simulink model "receiver"  (R2021b)
settings: Solver=VariableStepAuto  StartTime=0.0  StopTime=10000/3.2e6  RelTol=1e-3
PreLoadFcn:
  | setup_receiver
InitFcn:
  | setup_receiver
values from neighbouring files (symbols this model uses):
  fir_bbuf = reshape([fir_barker_13; fir_barker_13; fir_barker_13], [1, length(fir_barker_13)*3])    [setup_receiver.m]
  tx_data = [tx_data mbuf]    [setup_receiver.m]
undefined symbols (not defined in the file or in its folder): AXI4, designMultirateFIR, Lite, xlfda_numerator
libraries: hdlBasic x467, hdlsllib x15, dspmlti4 x8, hdlDSPIP x6, hdlSSR x6, dspswit3 x4, hdlUtilities x3, commrandsrc3 x2, dspsigops x2, simulink x1, vmcUtilities x1
(part 4 of 6)

== system receiver/QPSK System/RF-DAC ==
  note: Not Ready
  Data In : Inport
  Coarse Delay : Subsystem
  Interpolation Filter : Subsystem  mask{interp=8x}
      mask prompts: interp "Interpolation Factor:"
      mask init:
      | fir0 = dsp.FIRInterpolator('InterpolationFactor', 2,...
      |                            'CoefficientsDataType', 'Custom',...
      |                            'CustomCoefficientsDataType', numerictype([], 16, 14),...
      |                            'FullPrecisionOverride', false,...
      |                            'OutputDataType', 'Custom',...
      |                            'CustomOutputDataType', numerictype([], 16, 14),...
      |                            'Numerator', [-6, 0 54, 0, -254, 0, 1230, 2048, 1230, 0, -254, 0, 54, 0, -6]/(2048));
      | fir1 = dsp.FIRInterpolator('InterpolationFactor', 2,...
      |                            'CoefficientsDataType', 'Custom',...
      |                            'CustomCoefficientsDataType', numerictype([], 16, 14),...
      |                            'FullPrecisionOverride', false,...
      |                            'OutputDataType', 'Custom',...
      |                            'CustomOutputDataType', numerictype([], 16, 14),...
      |                            'Numerator', [-12, 0, 84, 0, -337, 0, 1008, 0, -2693, 0, 10142, 16384, 10142, 0, -2693, 0, 1008, 0, -337, 0, 84, 0 ,-12]/(16384));
      | fir2 = dsp.FIRInterpolator('InterpolationFactor', 2,...
      |                            'CoefficientsDataType', 'Custom',...
      |                            'CustomCoefficientsDataType', numerictype([], 16, 14),...
      |                            'FullPrecisionOverride', false,...
      |                            'OutputDataType', 'Custom',...
      |                            'CustomOutputDataType', numerictype([], 16, 14),...
      |                            'Numerator', [5, 0, -17, 0, 44, 0, -96, 0, 187, 0, -335, 0, 565, 0, -906, 0, 1401, 0, -2112, 0, 3145, 0, -4723, 0, 7415, 0, -13331, 0, 41526, 65536, 41526, 0, -13331, 0, 7415, 0, -4723, 0, 3145, 0, -2112, 0, 1401, 0, -906, 0, 565, 0, -335, 0, 187, 0, -96, 0, 44, 0, -17, 0, 5]/(65536));
      | switch get_param(gcb, 'interp')
      |     case '1x'
      |         if ~strcmp(get_param([gcb, '/FIR 0'], 'Commented'), 'through')
      |             set_param([gcb, '/FIR 0'],'Commented','through');
      |         end
      |         
      |         if ~strcmp(get_param([gcb, '/FIR 1'], 'Commented'), 'through')
      |             set_param([gcb, '/FIR 1'],'Commented','through');
      |         end
      |         
      |         if ~strcmp(get_param([gcb, '/FIR 2'], 'Commented'), 'through')
      |             set_param([gcb, '/FIR 2'],'Commented','through');
      |         end
      |             
      |     case '2x'
      |         if ~strcmp(get_param([gcb, '/FIR 0'], 'Commented'), 'through')
      |             set_param([gcb, '/FIR 0'],'Commented','through');
      |         end
      |         
      |         if ~strcmp(get_param([gcb, '/FIR 1'], 'Commented'), 'through')
      |             set_param([gcb, '/FIR 1'],'Commented','through');
      |         end
      |         
      |         if ~strcmp(get_param([gcb, '/FIR 2'], 'Commented'), 'off')
      |             set_param([gcb, '/FIR 2'],'Commented','off');
      |         end
      | 
      |     case '4x'
      |         if ~strcmp(get_param([gcb, '/FIR 0'], 'Commented'), 'through')
      |             set_param([gcb, '/FIR 0'],'Commented','through');
      |         end
      |         
      |         if ~strcmp(get_param([gcb, '/FIR 1'], 'Commented'), 'off')
      |             set_param([gcb, '/FIR 1'],'Commented','off');
      |         end
      |         
      |         if ~strcmp(get_param([gcb, '/FIR 2'], 'Commented'), 'off')
      |             set_param([gcb, '/FIR 2'],'Commented','off');
      |         end
      |         
      |     case '8x'
      |         if ~strcmp(get_param([gcb, '/FIR 0'], 'Commented'), 'off')
      |             set_param([gcb, '/FIR 0'],'Commented','off');
      |         end
      |         
      |         if ~strcmp(get_param([gcb, '/FIR 1'], 'Commented'), 'off')
      |             set_param([gcb, '/FIR 1'],'Commented','off');
      |         end
      |         
      |         if ~strcmp(get_param([gcb, '/FIR 2'], 'Commented'), 'off')
      |             set_param([gcb, '/FIR 2'],'Commented','off');
      |         end
      | 
      | end
      mask TypeOptions interp: 1x | 2x | 4x | 8x
      mask DialogControl DescGroupVar Prompt: RF-DAC Interpolation Filter
      mask DialogControl DescTextVar Prompt: This block simulates the RF-DAC interpolation stage using the same coefficients stored in the interpolation filters.
      mask DialogControl ParameterGroupVar Prompt: Main
  NCO and Mixer : Subsystem
  Output Filter : Subsystem
  QMC Gain & Phase : Subsystem
  QMC Threshold : Subsystem
  RF-DAC : Subsystem
  Data Out : Outport  VectorParamsAs1DForOutWhenUnconnected=off
  wires:
  RF-DAC/1(Data Out) -> Data Out/1
  QMC Threshold/1(Data Out) -> RF-DAC/1(Data In)
  Output Filter/1(Data Out) -> QMC Threshold/1(Data In)
  Coarse Delay/1(Data Out) -> Output Filter/1(Data In)
  QMC Gain & Phase/1(Data Out) -> Coarse Delay/1(Data In)
  Data In/1 -> Interpolation Filter/1(Data In)
  NCO and Mixer/1(Data Out) -> QMC Gain & Phase/1(Data In)
  Interpolation Filter/1(Data Out) -> NCO and Mixer/1(Data In)

== system receiver/Time Synchronisation/Loop Filter ==
  note: Get centre of symbol
  note: The input to the loop filter should only be changed once per symbol.
      |
      | Use an enable register with the strobe from the NCC to hold the data in place.
  note: Get centre of symbol
  Real In : Inport
  Imag In : Inport  Port=2
  Signal In : Inport  Port=3
  Valid In : Inport  Port=4
  Reset : Inport  Port=5
  AddSub : hdlBasic/AddSub  mode=Addition  use_carryin=off  use_carryout=off  en=off  latency=0  precision=User Defined  arith_type="Signed  (2's comp)"  n_bits=64  bin_pt=60  quantization=Truncate  overflow=Saturate  use_behavioral_HDL=off  hw_selection=Fabric  pipelined=off  XmcBlockStatus=1  maskContainerNames=tabcontainer1  block_type=addsub  block_config=sysgen:Addsub_config
  AddSub1 : hdlBasic/AddSub  mode=Addition  use_carryin=off  use_carryout=off  en=off  latency=0  precision=User Defined  arith_type="Signed  (2's comp)"  n_bits=64  bin_pt=60  quantization=Truncate  overflow=Saturate  use_behavioral_HDL=off  hw_selection=Fabric  pipelined=off  XmcBlockStatus=1  maskContainerNames=tabcontainer1  block_type=addsub  block_config=sysgen:Addsub_config
  Delay1 : hdlBasic/Delay  rst=off  en=off  latency=32/2  reg_retiming=off  XmcBlockStatus=1  maskContainerNames=group1  block_type=delay  block_config=sysgen:Delay_config
  Delay2 : hdlBasic/Delay  rst=off  en=off  latency=32/2  reg_retiming=off  XmcBlockStatus=1  maskContainerNames=group1  block_type=delay  block_config=sysgen:Delay_config
  Delay3 : hdlBasic/Delay  rst=off  en=off  latency=32/2  reg_retiming=off  XmcBlockStatus=1  maskContainerNames=group1  block_type=delay  block_config=sysgen:Delay_config
  K1_Gain : hdlBasic/CMult  const=K1  gui_display_data_type=Fixed-point  const_n_bits=32  const_bin_pt=30  float_type=Single  exp_bits=8  fraction_bits=24  en=off  latency=0  precision=Full  arith_type="Signed  (2's comp)"  n_bits=3+28+16  bin_pt=28+16  quantization=Truncate  overflow=Wrap  use_behavioral_HDL=off  mem_type=Distributed RAM  pipeline=off  XmcBlockStatus=1  maskContainerNames=tabcontainer1  block_type=cmult  block_config=sysgen:CMult_config
      settings: infoedit=[]
  K2_Gain : hdlBasic/CMult  const=K2  gui_display_data_type=Fixed-point  const_n_bits=32  const_bin_pt=30  float_type=Single  exp_bits=8  fraction_bits=24  en=off  latency=0  precision=Full  arith_type="Signed  (2's comp)"  n_bits=3+28+16  bin_pt=28+16  quantization=Truncate  overflow=Wrap  use_behavioral_HDL=off  mem_type=Distributed RAM  pipeline=off  XmcBlockStatus=1  maskContainerNames=tabcontainer1  block_type=cmult  block_config=sysgen:CMult_config
      settings: infoedit=[]
  Register : hdlBasic/Register  init=0  rst=on  en=on  XmcBlockStatus=1  maskContainerNames=tabcontainer1  block_type=register  block_config=sysgen:Register_config
  Register1 : hdlBasic/Register  init=0  rst=on  en=on  XmcBlockStatus=1  maskContainerNames=tabcontainer1  block_type=register  block_config=sysgen:Register_config
  Real Out : Outport  VectorParamsAs1DForOutWhenUnconnected=off
  Imag Out : Outport  Port=2  VectorParamsAs1DForOutWhenUnconnected=off
  Valid Out : Outport  Port=3  VectorParamsAs1DForOutWhenUnconnected=off
  Error Out : Outport  Port=4  VectorParamsAs1DForOutWhenUnconnected=off
  wires:
  Valid In/1 -> Register1/3, Delay3/1, Register/3
  AddSub1/1 -> Error Out/1
  Delay1/1 -> Real Out/1
  Delay2/1 -> Imag Out/1
  Register1/1 -> K2_Gain/1, K1_Gain/1
  Signal In/1 -> Register1/1
  Register/1 -> AddSub/2
  K1_Gain/1 -> AddSub1/1
  AddSub/1 -> AddSub1/2, Register/1
  Imag In/1 -> Delay2/1
  Real In/1 -> Delay1/1
  K2_Gain/1 -> AddSub/1
  Reset/1 -> Register1/2, Register/2
  Delay3/1 -> Valid Out/1

== system receiver/Time Synchronisation/NCC ==
  Error : Inport
  AddSub : hdlBasic/AddSub  mode=Addition  use_carryin=off  use_carryout=off  en=off  latency=0  precision=User Defined  arith_type=Unsigned  n_bits=n+f  bin_pt=f  quantization=Truncate  overflow=Wrap  use_behavioral_HDL=off  hw_selection=Fabric  pipelined=off  XmcBlockStatus=1  maskContainerNames=tabcontainer1  block_type=addsub  block_config=sysgen:Addsub_config
  AddSub1 : hdlBasic/AddSub  mode=Addition  use_carryin=off  use_carryout=off  en=off  latency=0  precision=User Defined  arith_type="Signed  (2's comp)"  n_bits=n+f  bin_pt=f  quantization=Truncate  overflow=Saturate  use_behavioral_HDL=off  hw_selection=Fabric  pipelined=off  XmcBlockStatus=1  maskContainerNames=tabcontainer1  block_type=addsub  block_config=sysgen:Addsub_config
  AddSub2 : hdlBasic/AddSub  mode=Subtraction  use_carryin=off  use_carryout=off  en=off  latency=0  precision=User Defined  arith_type="Signed  (2's comp)"  n_bits=n+f  bin_pt=f  quantization=Truncate  overflow=Flag as error  use_behavioral_HDL=off  hw_selection=Fabric  pipelined=off  XmcBlockStatus=1  maskContainerNames=tabcontainer1  block_type=addsub  block_config=sysgen:Addsub_config
  Constant : hdlBasic/Constant  const=1  gui_display_data_type=Fixed-point  arith_type=Unsigned  n_bits=1  bin_pt=0  preci_type=Single  exp_width=8  frac_width=24  explicit_period=off  period=1  XmcBlockStatus=1  maskContainerNames=tabcontainer1  block_type=constant  block_config=sysgen:Constant_config
  Constant1 : hdlBasic/Constant  const=r  gui_display_data_type=Fixed-point  arith_type=Unsigned  n_bits=n  bin_pt=0  preci_type=Single  exp_width=8  frac_width=24  explicit_period=off  period=1  XmcBlockStatus=1  maskContainerNames=tabcontainer1  block_type=constant  block_config=sysgen:Constant_config
  Mux : hdlBasic/Mux  inputs=2  en=off  latency=0  precision=Full  arith_type=Unsigned  n_bits=16  bin_pt=14  quantization=Truncate  overflow=Wrap  XmcBlockStatus=1  maskContainerNames=tabcontainer1  block_type=mux  block_config=sysgen:Mux_config
  Register : hdlBasic/Register  init=0  rst=off  en=off  XmcBlockStatus=1  maskContainerNames=tabcontainer1  block_type=register  block_config=sysgen:Register_config
  Relational : hdlBasic/Relational  mode=a>b  op_type=Bool  en=off  latency=0  XmcBlockStatus=1  maskContainerNames=tabcontainer1  block_type=relational  block_config=sysgen:Relational_config
  Relational1 : hdlBasic/Relational  mode=a>b  op_type=Bool  en=off  latency=0  XmcBlockStatus=1  maskContainerNames=tabcontainer1  block_type=relational  block_config=sysgen:Relational_config
  Strobe : Outport  VectorParamsAs1DForOutWhenUnconnected=off
  wires:
  Constant/1 -> AddSub1/1
  Error/1 -> AddSub1/2
  Relational/1 -> Strobe/1
  AddSub1/1 -> AddSub/2
  Mux/1 -> AddSub/1
  Relational1/1 -> Mux/1
  AddSub2/1 -> Mux/3
  Constant1/1 -> Relational1/2, AddSub2/2
  Register/1 -> Relational/1, Relational1/1, Mux/2, AddSub2/1
  AddSub/1 -> Register/1, Relational/2

== system receiver/Time Synchronisation/Timing Error Detector ==
  Real In : Inport
  Imag In : Inport  Port=2
  AddSub : hdlBasic/AddSub  mode=Subtraction  use_carryin=off  use_carryout=off  en=off  latency=0  precision=User Defined  arith_type="Signed  (2's comp)"  n_bits=31  bin_pt=30  quantization=Truncate  overflow=Saturate  use_behavioral_HDL=off  hw_selection=Fabric  pipelined=off  XmcBlockStatus=1  maskContainerNames=tabcontainer1  block_type=addsub  block_config=sysgen:Addsub_config
  AddSub1 : hdlBasic/AddSub  mode=Subtraction  use_carryin=off  use_carryout=off  en=off  latency=0  precision=User Defined  arith_type="Signed  (2's comp)"  n_bits=31  bin_pt=30  quantization=Truncate  overflow=Saturate  use_behavioral_HDL=off  hw_selection=Fabric  pipelined=off  XmcBlockStatus=1  maskContainerNames=tabcontainer1  block_type=addsub  block_config=sysgen:Addsub_config
  AddSub2 : hdlBasic/AddSub  mode=Addition  use_carryin=off  use_carryout=off  en=off  latency=0  precision=Full  arith_type="Signed  (2's comp)"  n_bits=16  bin_pt=13  quantization="Round  (unbiased: +/- Inf)"  overflow=Saturate  use_behavioral_HDL=off  hw_selection=Fabric  pipelined=off  XmcBlockStatus=1  maskContainerNames=tabcontainer1  block_type=addsub  block_config=sysgen:Addsub_config
  Delay : hdlBasic/Delay  rst=off  en=off  latency=32  reg_retiming=off  XmcBlockStatus=1  maskContainerNames=group1  block_type=delay  block_config=sysgen:Delay_config
  Delay1 : hdlBasic/Delay  rst=off  en=off  latency=32  reg_retiming=off  XmcBlockStatus=1  maskContainerNames=group1  block_type=delay  block_config=sysgen:Delay_config
  Mult1 : hdlBasic/Mult  precision=User Defined  arith_type=Unsigned  n_bits=31  bin_pt=30  quantization=Truncate  overflow=Saturate  en=off  latency=0  use_behavioral_HDL=off  opt=Speed  use_embedded=on  optimum_pipeline=off  pipeline=on  use_rpm=on  placement_style=Triangular  XmcBlockStatus=1  maskContainerNames=group1  block_type=mult  block_config=sysgen:Mult_config  block_width=598  block_height=876
  Mult2 : hdlBasic/Mult  precision=User Defined  arith_type=Unsigned  n_bits=31  bin_pt=30  quantization=Truncate  overflow=Saturate  en=off  latency=0  use_behavioral_HDL=off  opt=Speed  use_embedded=on  optimum_pipeline=off  pipeline=on  use_rpm=on  placement_style=Triangular  XmcBlockStatus=1  maskContainerNames=group1  block_type=mult  block_config=sysgen:Mult_config  block_width=598  block_height=876
  Reinterpret : hdlBasic/Reinterpret  force_arith_type=on  arith_type="Signed  (2's comp)"  force_bin_pt=on  bin_pt=15  XmcBlockStatus=1  maskContainerNames=group1  block_type=reinterpret  block_config=sysgen:Reinterpret_config
  Reinterpret1 : hdlBasic/Reinterpret  force_arith_type=on  arith_type="Signed  (2's comp)"  force_bin_pt=on  bin_pt=15  XmcBlockStatus=1  maskContainerNames=group1  block_type=reinterpret  block_config=sysgen:Reinterpret_config
  Error : Outport  VectorParamsAs1DForOutWhenUnconnected=off
  wires:
  AddSub2/1 -> Error/1
  Reinterpret1/1 -> Mult1/2, Mult1/1
  Reinterpret/1 -> Mult2/1, Mult2/2
  Delay/1 -> AddSub/2
  Mult1/1 -> Delay/1, AddSub/1
  AddSub1/1 -> AddSub2/2
  Mult2/1 -> AddSub1/1, Delay1/1
  Delay1/1 -> AddSub1/2
  AddSub/1 -> AddSub2/1
  Imag In/1 -> Reinterpret/1
  Real In/1 -> Reinterpret1/1

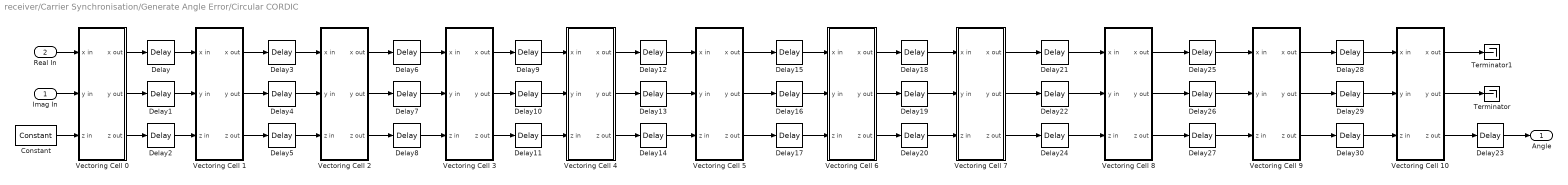
== system receiver/Carrier Synchronisation/Generate Angle Error/Circular CORDIC ==
  Imag In : Inport
  Real In : Inport  Port=2
  Constant : hdlBasic/Constant  const=0  gui_display_data_type=Fixed-point  arith_type=Signed (2's comp)  n_bits=16  bin_pt=14  preci_type=Single  exp_width=8  frac_width=24  explicit_period=off  period=1  XmcBlockStatus=1  maskContainerNames=tabcontainer1  block_type=constant  block_config=sysgen:Constant_config
  Delay{,1..30} (31 alike) : hdlBasic/Delay  rst=off  en=off  latency=1  reg_retiming=off  XmcBlockStatus=1  maskContainerNames=group1  block_type=delay  block_config=sysgen:Delay_config
  Terminator : Terminator
  Terminator1 : Terminator
  Vectoring Cell 0 : Subsystem  mask(Cordic Vectoring Cell){i=0}
      mask prompts: i "Iteration:"
      mask help: some notes to go here
      mask DialogControl DescGroupVar Prompt: CORDIC Vectoring Cell
      mask DialogControl DescTextVar Prompt: A single cell of a vectoring CORDIC unrolled architecture.
      mask DialogControl ParameterGroupVar Prompt: Main
  Vectoring Cell 1 : Subsystem  mask(Cordic Vectoring Cell){i=1}
      mask prompts: i "Iteration:"
      mask help: some notes to go here
      mask DialogControl DescGroupVar Prompt: CORDIC Vectoring Cell
      mask DialogControl DescTextVar Prompt: A single cell of a vectoring CORDIC unrolled architecture.
      mask DialogControl ParameterGroupVar Prompt: Main
  Vectoring Cell 10 : Subsystem  mask(Cordic Vectoring Cell){i=10}
      mask prompts: i "Iteration:"
      mask help: some notes to go here
      mask DialogControl DescGroupVar Prompt: CORDIC Vectoring Cell
      mask DialogControl DescTextVar Prompt: A single cell of a vectoring CORDIC unrolled architecture.
      mask DialogControl ParameterGroupVar Prompt: Main
  Vectoring Cell 2 : Subsystem  mask(Cordic Vectoring Cell){i=2}
      mask prompts: i "Iteration:"
      mask help: some notes to go here
      mask DialogControl DescGroupVar Prompt: CORDIC Vectoring Cell
      mask DialogControl DescTextVar Prompt: A single cell of a vectoring CORDIC unrolled architecture.
      mask DialogControl ParameterGroupVar Prompt: Main
  Vectoring Cell 3 : Subsystem  mask(Cordic Vectoring Cell){i=3}
      mask prompts: i "Iteration:"
      mask help: some notes to go here
      mask DialogControl DescGroupVar Prompt: CORDIC Vectoring Cell
      mask DialogControl DescTextVar Prompt: A single cell of a vectoring CORDIC unrolled architecture.
      mask DialogControl ParameterGroupVar Prompt: Main
  Vectoring Cell 4 : Subsystem  mask(Cordic Vectoring Cell){i=4}
      mask prompts: i "Iteration:"
      mask help: some notes to go here
      mask DialogControl DescGroupVar Prompt: CORDIC Vectoring Cell
      mask DialogControl DescTextVar Prompt: A single cell of a vectoring CORDIC unrolled architecture.
      mask DialogControl ParameterGroupVar Prompt: Main
  Vectoring Cell 5 : Subsystem  mask(Cordic Vectoring Cell){i=5}
      mask prompts: i "Iteration:"
      mask help: some notes to go here
      mask DialogControl DescGroupVar Prompt: CORDIC Vectoring Cell
      mask DialogControl DescTextVar Prompt: A single cell of a vectoring CORDIC unrolled architecture.
      mask DialogControl ParameterGroupVar Prompt: Main
  Vectoring Cell 6 : Subsystem  mask(Cordic Vectoring Cell){i=6}
      mask prompts: i "Iteration:"
      mask help: some notes to go here
      mask DialogControl DescGroupVar Prompt: CORDIC Vectoring Cell
      mask DialogControl DescTextVar Prompt: A single cell of a vectoring CORDIC unrolled architecture.
      mask DialogControl ParameterGroupVar Prompt: Main
  Vectoring Cell 7 : Subsystem  mask(Cordic Vectoring Cell){i=7}
      mask prompts: i "Iteration:"
      mask help: some notes to go here
      mask DialogControl DescGroupVar Prompt: CORDIC Vectoring Cell
      mask DialogControl DescTextVar Prompt: A single cell of a vectoring CORDIC unrolled architecture.
      mask DialogControl ParameterGroupVar Prompt: Main
  Vectoring Cell 8 : Subsystem  mask(Cordic Vectoring Cell){i=8}
      mask prompts: i "Iteration:"
      mask help: some notes to go here
      mask DialogControl DescGroupVar Prompt: CORDIC Vectoring Cell
      mask DialogControl DescTextVar Prompt: A single cell of a vectoring CORDIC unrolled architecture.
      mask DialogControl ParameterGroupVar Prompt: Main
  Vectoring Cell 9 : Subsystem  mask(Cordic Vectoring Cell){i=9}
      mask prompts: i "Iteration:"
      mask help: some notes to go here
      mask DialogControl DescGroupVar Prompt: CORDIC Vectoring Cell
      mask DialogControl DescTextVar Prompt: A single cell of a vectoring CORDIC unrolled architecture.
      mask DialogControl ParameterGroupVar Prompt: Main
  Angle : Outport  VectorParamsAs1DForOutWhenUnconnected=off
  wires:
  Delay23/1 -> Angle/1
  Constant/1 -> Vectoring Cell 0/3(z in)
  Imag In/1 -> Vectoring Cell 0/2(y in)
  Real In/1 -> Vectoring Cell 0/1(x in)
  Delay11/1 -> Vectoring Cell 4/3(z in)
  Delay17/1 -> Vectoring Cell 6/3(z in)
  Vectoring Cell 5/3(z out) -> Delay17/1
  Delay2/1 -> Vectoring Cell 1/3(z in)
  Vectoring Cell 4/1(x out) -> Delay12/1
  Vectoring Cell 4/2(y out) -> Delay13/1
  Delay12/1 -> Vectoring Cell 5/1(x in)
  Vectoring Cell 0/2(y out) -> Delay1/1
  Vectoring Cell 6/1(x out) -> Delay18/1
  Vectoring Cell 2/3(z out) -> Delay8/1
  Vectoring Cell 0/1(x out) -> Delay/1
  Vectoring Cell 5/2(y out) -> Delay16/1
  Delay/1 -> Vectoring Cell 1/1(x in)
  Vectoring Cell 5/1(x out) -> Delay15/1
  Vectoring Cell 1/2(y out) -> Delay4/1
  Vectoring Cell 3/2(y out) -> Delay10/1
  Delay8/1 -> Vectoring Cell 3/3(z in)
  Vectoring Cell 4/3(z out) -> Delay14/1
  Delay3/1 -> Vectoring Cell 2/1(x in)
  Delay4/1 -> Vectoring Cell 2/2(y in)
  Delay19/1 -> Vectoring Cell 7/2(y in)
  Delay6/1 -> Vectoring Cell 3/1(x in)
  Vectoring Cell 3/3(z out) -> Delay11/1
  Vectoring Cell 2/2(y out) -> Delay7/1
  Delay10/1 -> Vectoring Cell 4/2(y in)
  Vectoring Cell 0/3(z out) -> Delay2/1
  Delay18/1 -> Vectoring Cell 7/1(x in)
  Delay16/1 -> Vectoring Cell 6/2(y in)
  Vectoring Cell 1/1(x out) -> Delay3/1
  Delay9/1 -> Vectoring Cell 4/1(x in)
  Delay13/1 -> Vectoring Cell 5/2(y in)
  Vectoring Cell 3/1(x out) -> Delay9/1
  Delay1/1 -> Vectoring Cell 1/2(y in)
  Delay7/1 -> Vectoring Cell 3/2(y in)
  Delay15/1 -> Vectoring Cell 6/1(x in)
  Delay20/1 -> Vectoring Cell 7/3(z in)
  Delay14/1 -> Vectoring Cell 5/3(z in)
  Vectoring Cell 1/3(z out) -> Delay5/1
  Vectoring Cell 2/1(x out) -> Delay6/1
  Vectoring Cell 6/2(y out) -> Delay19/1
  Delay5/1 -> Vectoring Cell 2/3(z in)
  Vectoring Cell 6/3(z out) -> Delay20/1
  Vectoring Cell 7/1(x out) -> Delay21/1
  Vectoring Cell 7/2(y out) -> Delay22/1
  Vectoring Cell 7/3(z out) -> Delay24/1
  Delay22/1 -> Vectoring Cell 8/2(y in)
  Delay21/1 -> Vectoring Cell 8/1(x in)
  Delay24/1 -> Vectoring Cell 8/3(z in)
  Delay27/1 -> Vectoring Cell 9/3(z in)
  Delay25/1 -> Vectoring Cell 9/1(x in)
  Delay26/1 -> Vectoring Cell 9/2(y in)
  Vectoring Cell 8/1(x out) -> Delay25/1
  Vectoring Cell 8/2(y out) -> Delay26/1
  Vectoring Cell 8/3(z out) -> Delay27/1
  Delay29/1 -> Vectoring Cell 10/2(y in)
  Delay28/1 -> Vectoring Cell 10/1(x in)
  Delay30/1 -> Vectoring Cell 10/3(z in)
  Vectoring Cell 10/1(x out) -> Terminator1/1
  Vectoring Cell 10/2(y out) -> Terminator/1
  Vectoring Cell 10/3(z out) -> Delay23/1
  Vectoring Cell 9/1(x out) -> Delay28/1
  Vectoring Cell 9/2(y out) -> Delay29/1
  Vectoring Cell 9/3(z out) -> Delay30/1

== system receiver/Carrier Synchronisation/Generate NCO/Loop Filter ==
  Signal : Inport
  Strobe : Inport  Port=2
  Reset : Inport  Port=3
  AddSub : hdlBasic/AddSub  mode=Addition  use_carryin=off  use_carryout=off  en=off  latency=0  precision=User Defined  arith_type="Signed  (2's comp)"  n_bits=40  bin_pt=38  quantization=Truncate  overflow=Flag as error  use_behavioral_HDL=off  hw_selection=Fabric  pipelined=off  XmcBlockStatus=1  maskContainerNames=tabcontainer1  block_type=addsub  block_config=sysgen:Addsub_config
  AddSub1 : hdlBasic/AddSub  mode=Addition  use_carryin=off  use_carryout=off  en=off  latency=0  precision=User Defined  arith_type="Signed  (2's comp)"  n_bits=40  bin_pt=38  quantization=Truncate  overflow=Wrap  use_behavioral_HDL=off  hw_selection=Fabric  pipelined=off  XmcBlockStatus=1  maskContainerNames=tabcontainer1  block_type=addsub  block_config=sysgen:Addsub_config
  K1_Gain : hdlBasic/CMult  const=K1  gui_display_data_type=Fixed-point  const_n_bits=16  const_bin_pt=16  float_type=Single  exp_bits=8  fraction_bits=24  en=off  latency=0  precision=Full  arith_type="Signed  (2's comp)"  n_bits=20  bin_pt=14  quantization=Truncate  overflow=Wrap  use_behavioral_HDL=off  mem_type=Distributed RAM  pipeline=off  XmcBlockStatus=1  maskContainerNames=tabcontainer1  block_type=cmult  block_config=sysgen:CMult_config
      settings: infoedit=[]
  K2_Gain : hdlBasic/CMult  const=K2  gui_display_data_type=Fixed-point  const_n_bits=18  const_bin_pt=18  float_type=Single  exp_bits=8  fraction_bits=24  en=off  latency=0  precision=Full  arith_type="Signed  (2's comp)"  n_bits=20  bin_pt=14  quantization=Truncate  overflow=Wrap  use_behavioral_HDL=off  mem_type=Distributed RAM  pipeline=off  XmcBlockStatus=1  maskContainerNames=tabcontainer1  block_type=cmult  block_config=sysgen:CMult_config
      settings: infoedit=[]
  Register : hdlBasic/Register  init=0  rst=on  en=on  XmcBlockStatus=1  maskContainerNames=tabcontainer1  block_type=register  block_config=sysgen:Register_config
  Register1 : hdlBasic/Register  init=0  rst=on  en=on  XmcBlockStatus=1  maskContainerNames=tabcontainer1  block_type=register  block_config=sysgen:Register_config
  Register2 : hdlBasic/Register  init=0  rst=off  en=off  XmcBlockStatus=1  maskContainerNames=tabcontainer1  block_type=register  block_config=sysgen:Register_config
  Register3 : hdlBasic/Register  init=0  rst=off  en=off  XmcBlockStatus=1  maskContainerNames=tabcontainer1  block_type=register  block_config=sysgen:Register_config
  Register4 : hdlBasic/Register  init=0  rst=off  en=off  XmcBlockStatus=1  maskContainerNames=tabcontainer1  block_type=register  block_config=sysgen:Register_config
  Error : Outport  VectorParamsAs1DForOutWhenUnconnected=off
  Valid : Outport  Port=2  VectorParamsAs1DForOutWhenUnconnected=off
  wires:
  Strobe/1 -> Register1/3, Register2/1
  Register4/1 -> Valid/1
  Register3/1 -> Error/1
  K1_Gain/1 -> AddSub1/1
  AddSub1/1 -> Register3/1
  Register1/1 -> K1_Gain/1, K2_Gain/1
  Register/1 -> AddSub/2
  AddSub/1 -> Register/1, AddSub1/2
  K2_Gain/1 -> AddSub/1
  Signal/1 -> Register1/1
  Reset/1 -> Register1/2, Register/2
  Register2/1 -> Register/3, Register4/1

== system receiver/Carrier Synchronisation/Generate NCO/NCO ==
  Step Size : Inport
  En_in : Inport  Port=2
  AddSub4 : hdlBasic/AddSub  mode=Addition  use_carryin=off  use_carryout=off  en=off  latency=0  precision=User Defined  arith_type="Signed  (2's comp)"  n_bits=n+b  bin_pt=b  quantization=Truncate  overflow=Wrap  use_behavioral_HDL=off  hw_selection=Fabric  pipelined=off  XmcBlockStatus=1  maskContainerNames=tabcontainer1  block_type=addsub  block_config=sysgen:Addsub_config
  CMult1 : hdlBasic/CMult  const=(2^n)/(2*pi)  gui_display_data_type=Fixed-point  const_n_bits=k_n+b  const_bin_pt=b  float_type=Single  exp_bits=8  fraction_bits=24  en=off  latency=0  precision=User Defined  arith_type="Signed  (2's comp)"  n_bits=n+b  bin_pt=b  quantization=Truncate  overflow=Wrap  use_behavioral_HDL=off  mem_type=Distributed RAM  pipeline=off  XmcBlockStatus=1  maskContainerNames=tabcontainer1  block_type=cmult  block_config=sysgen:CMult_config
      settings: infoedit=[]
  Convert1 : hdlBasic/Convert  gui_display_data_type=Fixed-point  arith_type=Unsigned  n_bits=n  bin_pt=0  float_type=Single  exp_bits=8  fraction_bits=24  quantization=Truncate  overflow=Wrap  en=off  latency=0  pipeline=off  XmcBlockStatus=1  maskContainerNames=group2  block_type=convert  block_config=sysgen:Convert_config  block_width=595  block_height=885
  Cos ROM : hdlBasic/ROM  depth=2^n  initVector=cos(pi*(0:((2^n)-1))/(2^(n-1)))  distributed_mem=Block RAM  rst=off  init_reg=0  en=off  latency=1  gui_display_data_type=Fixed-point  arith_type="Signed  (2's comp)"  n_bits=18  bin_pt=16  preci_type=Single  exp_width=8  frac_width=24  optimize=Area  use_rpm=on  simulation_type=fast_sim  XmcBlockStatus=1  maskContainerNames=tabcontainer1  block_type=sprom  block_config=sysgen:SPROM_config
  Neg Sin ROM : hdlBasic/ROM  depth=2^n  initVector=-sin(pi*(0:((2^n)-1))/(2^(n-1)))  distributed_mem=Block RAM  rst=off  init_reg=0  en=off  latency=1  gui_display_data_type=Fixed-point  arith_type="Signed  (2's comp)"  n_bits=18  bin_pt=16  preci_type=Single  exp_width=8  frac_width=24  optimize=Area  use_rpm=on  simulation_type=fast_sim  XmcBlockStatus=1  maskContainerNames=tabcontainer1  block_type=sprom  block_config=sysgen:SPROM_config
  Register : hdlBasic/Register  init=0  rst=off  en=off  XmcBlockStatus=1  maskContainerNames=tabcontainer1  block_type=register  block_config=sysgen:Register_config
  Register1 : hdlBasic/Register  init=0  rst=off  en=on  XmcBlockStatus=1  maskContainerNames=tabcontainer1  block_type=register  block_config=sysgen:Register_config
  Cos : Outport  VectorParamsAs1DForOutWhenUnconnected=off
  Neg Sin : Outport  Port=2  VectorParamsAs1DForOutWhenUnconnected=off
  En_out : Outport  Port=3  VectorParamsAs1DForOutWhenUnconnected=off
  wires:
  Register/1 -> En_out/1
  Cos ROM/1 -> Cos/1
  En_in/1 -> Register1/2, Register/1
  Step Size/1 -> CMult1/1
  CMult1/1 -> AddSub4/1
  Register1/1 -> AddSub4/2
  Neg Sin ROM/1 -> Neg Sin/1
  AddSub4/1 -> Convert1/1, Register1/1
  Convert1/1 -> Cos ROM/1, Neg Sin ROM/1

== system receiver/Frame Synchronisation/BPSK Frame Sync/DBPSK Convert ==
  Data In : Inport
  Valid In : Inport  Port=2
  Constant : hdlBasic/Constant  const=1.0  gui_display_data_type=Fixed-point  arith_type=Signed (2's comp)  n_bits=2  bin_pt=0  preci_type=Single  exp_width=8  frac_width=24  explicit_period=off  period=1  XmcBlockStatus=1  maskContainerNames=tabcontainer1  block_type=constant  block_config=sysgen:Constant_config
  Constant1 : hdlBasic/Constant  const=-1.0  gui_display_data_type=Fixed-point  arith_type=Signed (2's comp)  n_bits=2  bin_pt=0  preci_type=Single  exp_width=8  frac_width=24  explicit_period=off  period=1  XmcBlockStatus=1  maskContainerNames=tabcontainer1  block_type=constant  block_config=sysgen:Constant_config
  Mux : hdlBasic/Mux  inputs=2  en=off  latency=0  precision=Full  arith_type=Unsigned  n_bits=16  bin_pt=14  quantization=Truncate  overflow=Wrap  XmcBlockStatus=1  maskContainerNames=tabcontainer1  block_type=mux  block_config=sysgen:Mux_config
  Data Out : Outport  VectorParamsAs1DForOutWhenUnconnected=off
  Valid Out : Outport  Port=2  VectorParamsAs1DForOutWhenUnconnected=off
  wires:
  Data In/1 -> Mux/1
  Valid In/1 -> Valid Out/1
  Mux/1 -> Data Out/1
  Constant1/1 -> Mux/3
  Constant/1 -> Mux/2

== system receiver/Frame Synchronisation/BPSK Frame Sync/DBPSK Decision ==
  Data In : Inport
  Valid In : Inport  Port=2
  Logical1 : hdlBasic/Logical  logical_function=XOR  inputs=2  en=off  latency=0  precision=Full  arith_type=Unsigned  n_bits=16  bin_pt=0  align_bp=on  overflow=[]  quantization=[]  XmcBlockStatus=1  maskContainerNames=tabcontainer1  block_type=logical  block_config=sysgen:Logical_config
  Register : hdlBasic/Register  init=0  rst=off  en=on  XmcBlockStatus=1  maskContainerNames=tabcontainer1  block_type=register  block_config=sysgen:Register_config
  Register2 : hdlBasic/Register  init=0  rst=off  en=off  XmcBlockStatus=1  maskContainerNames=tabcontainer1  block_type=register  block_config=sysgen:Register_config
  Register3 : hdlBasic/Register  init=0  rst=off  en=on  XmcBlockStatus=1  maskContainerNames=tabcontainer1  block_type=register  block_config=sysgen:Register_config
  Register4 : hdlBasic/Register  init=0  rst=off  en=on  XmcBlockStatus=1  maskContainerNames=tabcontainer1  block_type=register  block_config=sysgen:Register_config
  Register5 : hdlBasic/Register  init=0  rst=off  en=off  XmcBlockStatus=1  maskContainerNames=tabcontainer1  block_type=register  block_config=sysgen:Register_config
  Data Out : Outport  VectorParamsAs1DForOutWhenUnconnected=off
  Valid Out : Outport  Port=2  VectorParamsAs1DForOutWhenUnconnected=off
  wires:
  Data In/1 -> Register/1
  Register5/1 -> Valid Out/1
  Valid In/1 -> Register/2, Register2/1
  Register3/1 -> Logical1/1
  Register/1 -> Register3/1, Logical1/2
  Logical1/1 -> Register4/1
  Register2/1 -> Register3/2, Register5/1, Register4/2
  Register4/1 -> Data Out/1

== system receiver/Frame Synchronisation/BPSK Frame Sync/Rising Edge Detector ==
  Input : Inport
  Inverter : hdlBasic/Inverter  en=off  latency=0  XmcBlockStatus=1  maskContainerNames=group2  block_type=inv  block_config=sysgen:Inverter_config
  Logical1 : hdlBasic/Logical  logical_function=AND  inputs=2  en=off  latency=0  precision=Full  arith_type=Unsigned  n_bits=16  bin_pt=0  align_bp=on  overflow=[]  quantization=[]  XmcBlockStatus=1  maskContainerNames=tabcontainer1  block_type=logical  block_config=sysgen:Logical_config
  Register2 : hdlBasic/Register  init=0  rst=off  en=off  XmcBlockStatus=1  maskContainerNames=tabcontainer1  block_type=register  block_config=sysgen:Register_config
  Output : Outport  VectorParamsAs1DForOutWhenUnconnected=off
  wires:
  Register2/1 -> Inverter/1
  Inverter/1 -> Logical1/1
  Input/1 -> Register2/1, Logical1/2
  Logical1/1 -> Output/1

== system receiver/Frame Synchronisation/BPSK Frame Sync/Shift Register ==
  Data In : Inport
  Valid In : Inport  Port=2
  Concat : hdlBasic/Concat  num_inputs=8  XmcBlockStatus=1  maskContainerNames=group1  block_type=concat  block_config=sysgen:Concat_config
  Constant : hdlBasic/Constant  const=8  gui_display_data_type=Fixed-point  arith_type=Unsigned  n_bits=4  bin_pt=0  preci_type=Single  exp_width=8  frac_width=24  explicit_period=off  period=1  XmcBlockStatus=1  maskContainerNames=tabcontainer1  block_type=constant  block_config=sysgen:Constant_config
  Counter : hdlBasic/Counter  cnt_type=Count limited  cnt_to=8  operation=Up  start_count=0  cnt_by_val=1  arith_type=Unsigned  n_bits=4  bin_pt=0  load_pin=off  rst=on  en=on  explicit_period=Inferred from inputs  period=1  use_behavioral_HDL=off  implementation=Fabric  XmcBlockStatus=1  maskContainerNames=group1  block_type=counter  block_config=sysgen:Counter_config  block_width=531  block_height=1023
  Register{,1..7} (8 alike) : hdlBasic/Register  init=0  rst=off  en=on  XmcBlockStatus=1  maskContainerNames=tabcontainer1  block_type=register  block_config=sysgen:Register_config
  Relational : hdlBasic/Relational  mode=a=b  op_type=Bool  en=off  latency=0  XmcBlockStatus=1  maskContainerNames=tabcontainer1  block_type=relational  block_config=sysgen:Relational_config
  Data Out : Outport  VectorParamsAs1DForOutWhenUnconnected=off
  Valid Out : Outport  Port=2  VectorParamsAs1DForOutWhenUnconnected=off
  wires:
  Register/1 -> Concat/8
  Valid In/1 -> Counter/2, Register6/2, Register5/2, Register4/2, Register3/2, Register2/2, Register1/2, Register/2, Register7/2
  Register1/1 -> Concat/7, Register/1
  Register3/1 -> Concat/5, Register2/1
  Register6/1 -> Concat/2, Register5/1
  Register2/1 -> Concat/6, Register1/1
  Register7/1 -> Concat/1, Register6/1
  Register4/1 -> Concat/4, Register3/1
  Register5/1 -> Concat/3, Register4/1
  Data In/1 -> Register7/1
  Concat/1 -> Data Out/1
  Counter/1 -> Relational/1
  Constant/1 -> Relational/2
  Relational/1 -> Counter/1, Valid Out/1

== system receiver/Frame Synchronisation/QPSK Frame Sync/DQPSK Convert ==
  Data In : Inport
  Valid In : Inport  Port=2
  Constant : hdlBasic/Constant  const=1.0  gui_display_data_type=Fixed-point  arith_type=Signed (2's comp)  n_bits=2  bin_pt=0  preci_type=Single  exp_width=8  frac_width=24  explicit_period=off  period=1  XmcBlockStatus=1  maskContainerNames=tabcontainer1  block_type=constant  block_config=sysgen:Constant_config
  Constant1 : hdlBasic/Constant  const=-1.0  gui_display_data_type=Fixed-point  arith_type=Signed (2's comp)  n_bits=2  bin_pt=0  preci_type=Single  exp_width=8  frac_width=24  explicit_period=off  period=1  XmcBlockStatus=1  maskContainerNames=tabcontainer1  block_type=constant  block_config=sysgen:Constant_config
  Mux : hdlBasic/Mux  inputs=2  en=off  latency=0  precision=Full  arith_type=Unsigned  n_bits=16  bin_pt=14  quantization=Truncate  overflow=Wrap  XmcBlockStatus=1  maskContainerNames=tabcontainer1  block_type=mux  block_config=sysgen:Mux_config
  Data Out : Outport  VectorParamsAs1DForOutWhenUnconnected=off
  Valid Out : Outport  Port=2  VectorParamsAs1DForOutWhenUnconnected=off
  wires:
  Constant/1 -> Mux/2
  Constant1/1 -> Mux/3
  Mux/1 -> Data Out/1
  Valid In/1 -> Valid Out/1
  Data In/1 -> Mux/1

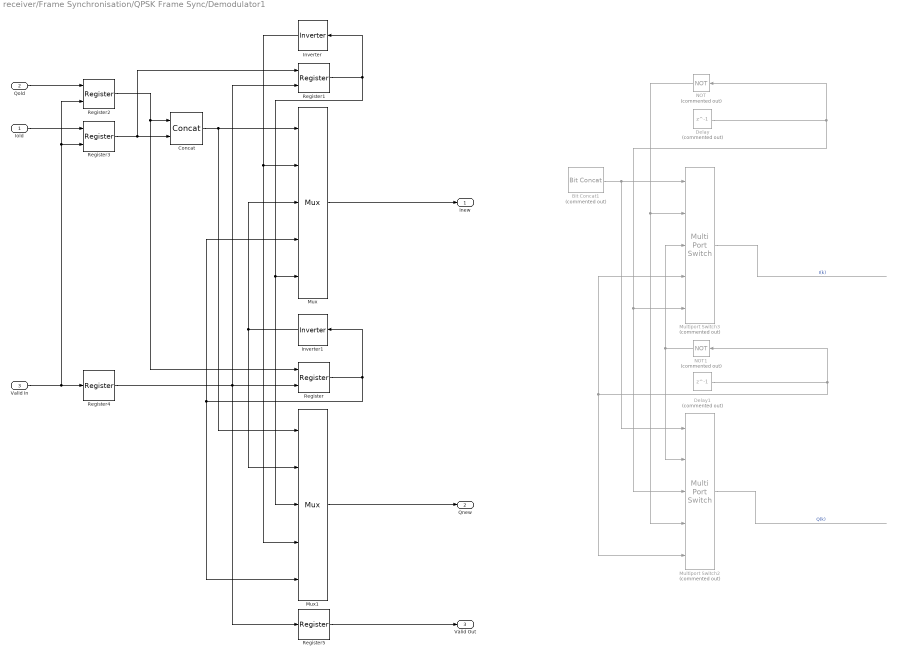
== system receiver/Frame Synchronisation/QPSK Frame Sync/Demodulator1 ==
  Iold : Inport
  Qold : Inport  Port=2
  Valid In : Inport  Port=3
  Bit Concat1 : hdlsllib/Logic and Bit Operations/Bit Concat  Commented=on  numInputs=2
  Concat : hdlBasic/Concat  num_inputs=2  XmcBlockStatus=1  maskContainerNames=group1  block_type=concat  block_config=sysgen:Concat_config
  Delay : Delay  Commented=on  DelayLength=1  ShowEnablePort=on
      settings: InputPortMap=u0,e6
  Delay1 : Delay  Commented=on  DelayLength=1  ShowEnablePort=on
      settings: InputPortMap=u0,e6
  Inverter : hdlBasic/Inverter  en=off  latency=0  XmcBlockStatus=1  maskContainerNames=group2  block_type=inv  block_config=sysgen:Inverter_config
  Inverter1 : hdlBasic/Inverter  en=off  latency=0  XmcBlockStatus=1  maskContainerNames=group2  block_type=inv  block_config=sysgen:Inverter_config
  Multiport Switch2 : MultiPortSwitch  Commented=on  DataPortOrder=Zero-based contiguous  Inputs=4  zeroidx=on
  Multiport Switch3 : MultiPortSwitch  Commented=on  DataPortOrder=Zero-based contiguous  Inputs=4  zeroidx=on
  Mux : hdlBasic/Mux  inputs=4  en=off  latency=1  precision=Full  arith_type=Unsigned  n_bits=16  bin_pt=14  quantization=Truncate  overflow=Wrap  XmcBlockStatus=1  maskContainerNames=tabcontainer1  block_type=mux  block_config=sysgen:Mux_config
  Mux1 : hdlBasic/Mux  inputs=4  en=off  latency=1  precision=Full  arith_type=Unsigned  n_bits=16  bin_pt=14  quantization=Truncate  overflow=Wrap  XmcBlockStatus=1  maskContainerNames=tabcontainer1  block_type=mux  block_config=sysgen:Mux_config
  NOT : Logic  Commented=on  Operator=NOT  IconShape=distinctive  AllPortsSameDT=off  OutDataTypeStr=boolean
  NOT1 : Logic  Commented=on  Operator=NOT  IconShape=distinctive  AllPortsSameDT=off  OutDataTypeStr=boolean
  Register{,1..3} (4 alike) : hdlBasic/Register  init=0  rst=off  en=on  XmcBlockStatus=1  maskContainerNames=tabcontainer1  block_type=register  block_config=sysgen:Register_config
  Register4 : hdlBasic/Register  init=0  rst=off  en=off  XmcBlockStatus=1  maskContainerNames=tabcontainer1  block_type=register  block_config=sysgen:Register_config
  Register5 : hdlBasic/Register  init=0  rst=off  en=off  XmcBlockStatus=1  maskContainerNames=tabcontainer1  block_type=register  block_config=sysgen:Register_config
  Inew : Outport
  Qnew : Outport  Port=2
  Valid Out : Outport  Port=3
  wires:
  ? -> Bit Concat1/1, Delay1/1
  Multiport Switch2/1 -> ?  "Q(k)"
  ? -> Delay/2, Delay1/2
  NOT/1 -> Multiport Switch2/4, Multiport Switch3/2
  Multiport Switch3/1 -> ?  "I(k)"
  Delay1/1 -> Multiport Switch3/4, Multiport Switch2/5, NOT1/1
  Bit Concat1/1 -> Multiport Switch3/1, Multiport Switch2/1
  ? -> Bit Concat1/2, Delay/1
  Delay/1 -> Multiport Switch2/3, Multiport Switch3/5, NOT/1
  NOT1/1 -> Multiport Switch3/3, Multiport Switch2/2
  Register5/1 -> Valid Out/1
  Register4/1 -> Register1/2, Register/2, Register5/1
  Register3/1 -> Register1/1, Concat/2
  Register2/1 -> Register/1, Concat/1
  Iold/1 -> Register3/1
  Qold/1 -> Register2/1
  Valid In/1 -> Register4/1, Register3/2, Register2/2
  Concat/1 -> Mux1/1, Mux/1
  Register1/1 -> Inverter/1, Mux/5, Mux1/3
  Mux/1 -> Inew/1
  Inverter/1 -> Mux1/4, Mux/2
  Mux1/1 -> Qnew/1
  Register/1 -> Inverter1/1, Mux1/5, Mux/4
  Inverter1/1 -> Mux/3, Mux1/2

== system receiver/Frame Synchronisation/QPSK Frame Sync/Rising Edge Detector ==
  Input : Inport
  Inverter : hdlBasic/Inverter  en=off  latency=0  XmcBlockStatus=1  maskContainerNames=group2  block_type=inv  block_config=sysgen:Inverter_config
  Logical1 : hdlBasic/Logical  logical_function=AND  inputs=2  en=off  latency=0  precision=Full  arith_type=Unsigned  n_bits=16  bin_pt=0  align_bp=on  overflow=[]  quantization=[]  XmcBlockStatus=1  maskContainerNames=tabcontainer1  block_type=logical  block_config=sysgen:Logical_config
  Register2 : hdlBasic/Register  init=0  rst=off  en=off  XmcBlockStatus=1  maskContainerNames=tabcontainer1  block_type=register  block_config=sysgen:Register_config
  Output : Outport  VectorParamsAs1DForOutWhenUnconnected=off
  wires:
  Register2/1 -> Inverter/1
  Inverter/1 -> Logical1/1
  Input/1 -> Register2/1, Logical1/2
  Logical1/1 -> Output/1

== system receiver/Frame Synchronisation/QPSK Frame Sync/Shift Register ==
  Data In : Inport
  Valid In : Inport  Port=2
  Concat : hdlBasic/Concat  num_inputs=4  XmcBlockStatus=1  maskContainerNames=group1  block_type=concat  block_config=sysgen:Concat_config
  Constant : hdlBasic/Constant  const=4  gui_display_data_type=Fixed-point  arith_type=Unsigned  n_bits=3  bin_pt=0  preci_type=Single  exp_width=8  frac_width=24  explicit_period=off  period=1  XmcBlockStatus=1  maskContainerNames=tabcontainer1  block_type=constant  block_config=sysgen:Constant_config
  Counter : hdlBasic/Counter  cnt_type=Count limited  cnt_to=4  operation=Up  start_count=0  cnt_by_val=1  arith_type=Unsigned  n_bits=3  bin_pt=0  load_pin=off  rst=on  en=on  explicit_period=Inferred from inputs  period=1  use_behavioral_HDL=off  implementation=Fabric  XmcBlockStatus=1  maskContainerNames=group1  block_type=counter  block_config=sysgen:Counter_config  block_width=531  block_height=1023
  Register{4..7} (4 alike) : hdlBasic/Register  init=0  rst=off  en=on  XmcBlockStatus=1  maskContainerNames=tabcontainer1  block_type=register  block_config=sysgen:Register_config
  Relational : hdlBasic/Relational  mode=a=b  op_type=Bool  en=off  latency=0  XmcBlockStatus=1  maskContainerNames=tabcontainer1  block_type=relational  block_config=sysgen:Relational_config
  Data Out : Outport  VectorParamsAs1DForOutWhenUnconnected=off
  Valid Out : Outport  Port=2  VectorParamsAs1DForOutWhenUnconnected=off
  wires:
  Valid In/1 -> Counter/2, Register6/2, Register5/2, Register4/2, Register7/2
  Register6/1 -> Concat/2, Register5/1
  Register7/1 -> Concat/1, Register6/1
  Register4/1 -> Concat/4
  Register5/1 -> Concat/3, Register4/1
  Data In/1 -> Register7/1
  Concat/1 -> Data Out/1
  Counter/1 -> Relational/1
  Constant/1 -> Relational/2
  Relational/1 -> Counter/1, Valid Out/1

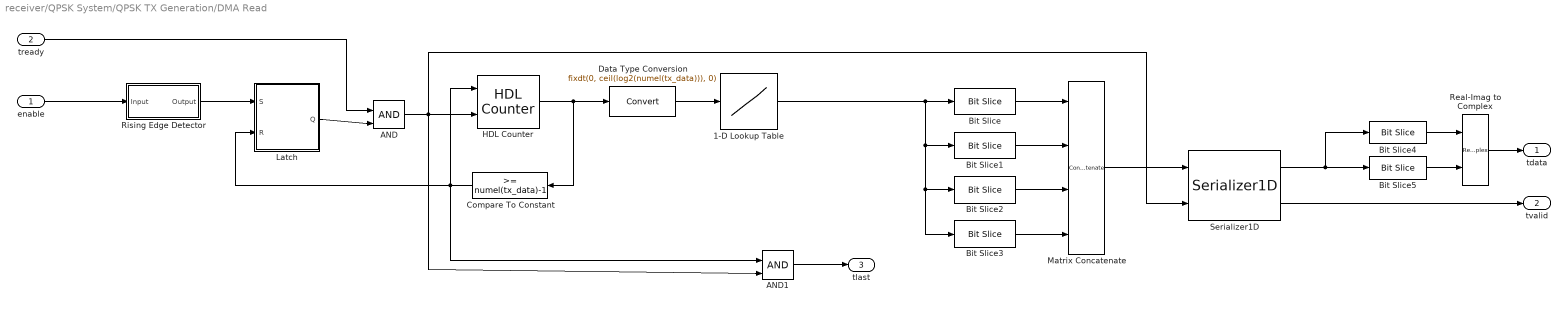
== system receiver/QPSK System/QPSK TX Generation/DMA Read ==
  enable : Inport
  tready : Inport  Port=2
  1-D Lookup Table : Lookup_n-D  NumberOfTableDimensions=1  BreakpointsForDimension1=[0:1:numel(tx_data)-1]  Table=tx_data  TableDataTypeStr=Inherit: Inherit from 'Table data'  ExtrapMethod=Clip  InternalRulePriority=Speed  OutDataTypeStr=Inherit: Inherit from 'Table data'  RndMeth=Simplest  InputSameDT=on
  AND : Logic  IconShape=distinctive  AllPortsSameDT=off  OutDataTypeStr=boolean
  AND1 : Logic  IconShape=distinctive  AllPortsSameDT=off  OutDataTypeStr=boolean
  Bit Slice : hdlsllib/Logic and Bit Operations/Bit Slice  lidx=1  ridx=0
      settings: SourceProductBaseCode=SL
  Bit Slice1 : hdlsllib/Logic and Bit Operations/Bit Slice  lidx=3  ridx=2
      settings: SourceProductBaseCode=SL
  Bit Slice2 : hdlsllib/Logic and Bit Operations/Bit Slice  lidx=5  ridx=4
      settings: SourceProductBaseCode=SL
  Bit Slice3 : hdlsllib/Logic and Bit Operations/Bit Slice  lidx=7  ridx=6
      settings: SourceProductBaseCode=SL
  Bit Slice4 : hdlsllib/Logic and Bit Operations/Bit Slice  lidx=0  ridx=0
      settings: SourceProductBaseCode=SL
  Bit Slice5 : hdlsllib/Logic and Bit Operations/Bit Slice  lidx=1  ridx=1
      settings: SourceProductBaseCode=SL
  Compare To Constant : simulink/Logic and Bit Operations/Compare To Constant  relop=>=  const=numel(tx_data)-1  OutDataTypeStr=boolean
  Data Type Conversion : DataTypeConversion  OutDataTypeStr=fixdt(0, ceil(log2(numel(tx_data))), 0)
  HDL Counter : hdlsllib/Sources/HDL Counter  CountType=Free running  CountInit=0  CountStep=1  CountMax=25  CountFromType=Initial value  CountFrom=0  CountResetPort=on  CountLoadPort=off  CountEnbPort=on  CountDirPort=off  CountHitOutputPort=off  CountDataType=Unsigned  CountWordLen=32  CountFracLen=0  CountSampTime=1
  Latch : Subsystem
  Matrix Concatenate : Concatenate  NumInputs=4  Mode=Multidimensional array  ConcatenateDimension=2
  Real-Imag to Complex : RealImagToComplex
  Rising Edge Detector : Subsystem
  Serializer1D : hdlsllib/HDL Operations/Serializer1D  Ratio=4  IdleCycles=0  validIn=on  startOut=off  validOut=on  inputDataDimensions=-1  inputSampleTime=-1  inputSignalType=auto
      settings: SourceProductBaseCode=SL
  tdata : Outport  VectorParamsAs1DForOutWhenUnconnected=off
  tvalid : Outport  Port=2  VectorParamsAs1DForOutWhenUnconnected=off
  tlast : Outport  Port=3  VectorParamsAs1DForOutWhenUnconnected=off
  wires:
  Serializer1D/2 -> tvalid/1
  1-D Lookup Table/1 -> Bit Slice/1, Bit Slice1/1, Bit Slice2/1, Bit Slice3/1
  Bit Slice2/1 -> Matrix Concatenate/3
  Bit Slice1/1 -> Matrix Concatenate/2
  Bit Slice3/1 -> Matrix Concatenate/4
  Bit Slice/1 -> Matrix Concatenate/1
  Matrix Concatenate/1 -> Serializer1D/1
  Compare To Constant/1 -> AND1/1, HDL Counter/1, Latch/2(R)
  enable/1 -> Rising Edge Detector/1(Input)
  HDL Counter/1 -> Compare To Constant/1, Data Type Conversion/1
  Data Type Conversion/1 -> 1-D Lookup Table/1
  Rising Edge Detector/1(Output) -> Latch/1(S)
  AND/1 -> AND1/2, Serializer1D/2, HDL Counter/2
  Latch/1(Q) -> AND/2
  tready/1 -> AND/1
  AND1/1 -> tlast/1
  Bit Slice4/1 -> Real-Imag to Complex/1
  Bit Slice5/1 -> Real-Imag to Complex/2
  Real-Imag to Complex/1 -> tdata/1
  Serializer1D/1 -> Bit Slice5/1, Bit Slice4/1

== system receiver/QPSK System/QPSK TX Generation/DQPSK Modulator ==
  Input : Inport
  Bit Concat : hdlsllib/Logic and Bit Operations/Bit Concat  numInputs=2
  Complex to Real-Imag : ComplexToRealImag
  Constant : Constant  Value=fi(1, 1, 16, 14)  OutDataTypeStr=fixdt(1,16,14)  SampleTime=-1
  Constant1 : Constant  Value=fi(-1, 1, 16, 14)  OutDataTypeStr=fixdt(1,16,14)  SampleTime=-1
  Constant2 : Constant  Value=fi(1, 1, 16, 14)  OutDataTypeStr=fixdt(1,16,14)  SampleTime=-1
  Constant3 : Constant  Value=fi(-1, 1, 16, 14)  OutDataTypeStr=fixdt(1,16,14)  SampleTime=-1
  Data Type Conversion : DataTypeConversion  OutDataTypeStr=boolean  RndMeth=Round
  Data Type Conversion1 : DataTypeConversion  OutDataTypeStr=boolean  RndMeth=Round
  Modulator : Subsystem
  Multiport Switch : MultiPortSwitch  DataPortOrder=Zero-based contiguous  Inputs=2  zeroidx=on
  Multiport Switch1 : MultiPortSwitch  DataPortOrder=Zero-based contiguous  Inputs=2  zeroidx=on
  Real-Imag to Complex : RealImagToComplex
  Output : Outport  VectorParamsAs1DForOutWhenUnconnected=off
  wires:
  Modulator/1(I(k)) -> Multiport Switch/1
  Modulator/2(Q(k)) -> Multiport Switch1/1
  Bit Concat/1 -> Modulator/1(IQ)
  Data Type Conversion/1 -> Bit Concat/2  "Q_new"
  Data Type Conversion1/1 -> Bit Concat/1  "P_new"
  Real-Imag to Complex/1 -> Output/1
  Multiport Switch/1 -> Real-Imag to Complex/1
  Constant1/1 -> Multiport Switch/3
  Constant/1 -> Multiport Switch/2
  Complex to Real-Imag/1 -> Data Type Conversion/1
  Input/1 -> Complex to Real-Imag/1
  Complex to Real-Imag/2 -> Data Type Conversion1/1
  Constant2/1 -> Multiport Switch1/2
  Constant3/1 -> Multiport Switch1/3
  Multiport Switch1/1 -> Real-Imag to Complex/2
